simulink model "part1_1_m2"  (R2019b)
settings: Solver=VariableStepAuto  StartTime=0.0  StopTime=1  RelTol=1e-3
settings Model: Creator=SEFA  LastModifiedBy=SEFA

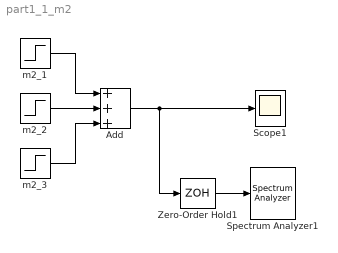
== system part1_1_m2 ==
  Add : Sum  Inputs=+++
  Scope1 : Scope
  Spectrum Analyzer1 : SpectrumAnalyzer
  Zero-Order Hold1 : ZeroOrderHold  SampleTime=1/2000
  m2_1 : Step  Time=0  SampleTime=1/100000
  "m2_2 " : Step  Time=0.05  After=-3  SampleTime=1/100000
  "m2_3 " : Step  Time=0.1  After=2  SampleTime=1/100000
  wires:
  Zero-Order Hold1/1 -> Spectrum Analyzer1/1
  Add/1 -> Zero-Order Hold1/1, Scope1/1
  m2_1/1 -> Add/1
  "m2_3 "/1 -> Add/3
  "m2_2 "/1 -> Add/2
